simulink model "LCK"  (R2018b)
settings: Solver=FixedStepDiscrete  StartTime=0.0  StopTime=inf  FixedStep=0.01  RelTol=1e-3
PostLoadFcn:
  | if any(exist('dsrtsu_mdlpostloadfcn', 'file') ~= 0), dsrtsu_mdlpostloadfcn('Execute', bdroot); end
values from neighbouring files (symbols this model uses):
  C_DEG2RAD = 0.0175    [LCK_Macro.sldd]
  C_KPH2MPS = 0.2778    [LCK_Macro.sldd]
  C_NEARZERO = 0.0001    [LCK_Macro.sldd]
  C_ONE = 1.0    [LCK_Macro.sldd]
  C_RAD2DEG = 57.2958    [LCK_Macro.sldd]
  C_ZERO = 0.0    [LCK_Macro.sldd]
  k_accel_pedal_pos_per_speed_x : value not decoded    [LCK_LogicPara.sldd]
  k_accel_pedal_pos_per_speed_z : value not decoded    [LCK_LogicPara.sldd]
  k_brake_suprress_hold = 1000.0    [LCK_LogicPara.sldd]
  k_driver_appl_torque_filt = 50.0    [LCK_LogicPara.sldd]
  k_driver_suppression_hold_time = 3000.0    [LCK_LogicPara.sldd]
  k_hands_on_wheel_hold_msec = 500.0    [LCK_LogicPara.sldd]
  k_hands_on_wheel_torque_hi = 0.2    [LCK_LogicPara.sldd]
  k_hands_on_wheel_torque_lo = 0.15    [LCK_LogicPara.sldd]
  k_handsoff_delay_cycles = 50.0    [LCK_LogicPara.sldd]
  k_handsoff_torq_Lo_CR = 0.3    [LCK_LogicPara.sldd]
  k_handson_delay_cycles = 5.0    [LCK_LogicPara.sldd]
  k_HighAccel_suppress_hold = 3000.0    [LCK_LogicPara.sldd]
  k_HLR_suprress_hold = 3000.0    [LCK_LogicPara.sldd]
  k_hs_StrAng_CR_threshold_z : value not decoded    [LCK_LogicPara.sldd]
  k_LC_Exit_Switch = 0.0    [LCK_LogicPara.sldd]
  k_LCG_Configured = 1.0    [LCK_LogicPara.sldd]
  k_LCK_A0_Rdy2Act_UseConst = 0.0    [LCK_LogicPara.sldd]
  k_LCK_A0Fac_ActSta : value not decoded    [LCK_CtrlPara.sldd]
  k_LCK_A0Fac_DrvStm : value not decoded    [LCK_CtrlPara.sldd]
  k_LCK_A0Shift_LftCurv : value not decoded    [LCK_CtrlPara.sldd]
  k_LCK_A0Shift_RgtCurv : value not decoded    [LCK_CtrlPara.sldd]
  k_LCK_A0Shift_StraLan = 0.0    [LCK_CtrlPara.sldd]
  k_LCK_A0ShiftFac_Dy_LftCurv : value not decoded    [LCK_CtrlPara.sldd]
  k_LCK_A0ShiftFac_Dy_RgtCurv : value not decoded    [LCK_CtrlPara.sldd]
  k_LCK_A0ShiftFac_Vspd : value not decoded    [LCK_CtrlPara.sldd]
  k_LCK_accel_inhibit_thold = 35.0    [LCK_LogicPara.sldd]
  k_LCK_Active2Ready_Mask = 255.0    [LCK_LogicPara.sldd]
  k_LCK_CvatRateBks : value not decoded    [LCK_CtrlPara.sldd]
  k_LCK_CvatrBks : value not decoded    [LCK_CtrlPara.sldd]
  k_LCK_DFac_Dy : value not decoded    [LCK_CtrlPara.sldd]
  k_LCK_DFac_Dy_Curv : value not decoded    [LCK_CtrlPara.sldd]
  k_LCK_DFac_HaCurCen : value not decoded    [LCK_CtrlPara.sldd]
  k_LCK_DFac_HaCurSid : value not decoded    [LCK_CtrlPara.sldd]
  k_LCK_DFac_HadCurCen : value not decoded    [LCK_CtrlPara.sldd]
  k_LCK_DFac_HadCurSid : value not decoded    [LCK_CtrlPara.sldd]
  k_LCK_DFac_HadStrCen : value not decoded    [LCK_CtrlPara.sldd]
  k_LCK_DFac_HadStrSid : value not decoded    [LCK_CtrlPara.sldd]
  k_LCK_DFac_HaStrCen : value not decoded    [LCK_CtrlPara.sldd]
  k_LCK_DFac_HaStrSid : value not decoded    [LCK_CtrlPara.sldd]
  k_LCK_DFac_Rad : value not decoded    [LCK_CtrlPara.sldd]
  k_LCK_DFac_SA_CurCen : value not decoded    [LCK_CtrlPara.sldd]
  k_LCK_DFac_SA_CurSid : value not decoded    [LCK_CtrlPara.sldd]
  k_LCK_DFac_SA_StrCen : value not decoded    [LCK_CtrlPara.sldd]
  k_LCK_DFac_SA_StrSid : value not decoded    [LCK_CtrlPara.sldd]
  k_LCK_DFac_SS_CurCen : value not decoded    [LCK_CtrlPara.sldd]
  k_LCK_DFac_SS_CurSid : value not decoded    [LCK_CtrlPara.sldd]
  k_LCK_DFac_SS_StrCen : value not decoded    [LCK_CtrlPara.sldd]
  k_LCK_DFac_SS_StrSid : value not decoded    [LCK_CtrlPara.sldd]
  k_LCK_DFac_Vspd : value not decoded    [LCK_CtrlPara.sldd]
  k_LCK_DlyTm_DrvStim = 0.2    [LCK_CtrlPara.sldd]
  k_LCK_DTermMax = 2.0    [LCK_CtrlPara.sldd]
  k_LCK_DyBks_Curv : value not decoded    [LCK_CtrlPara.sldd]
  k_LCK_Enable_POOnly = 1.0    [LCK_LogicPara.sldd]
  k_LCK_Entry_DistBuffer = 0.1    [LCK_LogicPara.sldd]
  k_LCK_Fac_Vspd2RngThr_FalRec = 0.23    [LCK_CtrlPara.sldd]
  k_LCK_Ffw_CvatSwh = 0.0    [LCK_CtrlPara.sldd]
  k_LCK_Ffw_DyBks : value not decoded    [LCK_CtrlPara.sldd]
  k_LCK_Ffw_TimCon_CmdFlt = 0.0    [LCK_CtrlPara.sldd]
  k_LCK_FfwDeltaFac_Rad_Lft : value not decoded    [LCK_CtrlPara.sldd]
  k_LCK_FfwDeltaFac_Rad_Rgt : value not decoded    [LCK_CtrlPara.sldd]
  k_LCK_FfwDeltaFac_Vspd : value not decoded    [LCK_CtrlPara.sldd]
  k_LCK_FfwFac_CvatRate_Lft : value not decoded    [LCK_CtrlPara.sldd]
  k_LCK_FfwFac_CvatRate_Rgt : value not decoded    [LCK_CtrlPara.sldd]
  k_LCK_FfwFac_Dy : value not decoded    [LCK_CtrlPara.sldd]
  k_LCK_FfwFac_Rad_Lft : value not decoded    [LCK_CtrlPara.sldd]
  k_LCK_FfwFac_Rad_Rgt : value not decoded    [LCK_CtrlPara.sldd]
  k_LCK_FfwFac_Vspd : value not decoded    [LCK_CtrlPara.sldd]
  k_LCK_FfwTorq_Cvat : value not decoded    [LCK_CtrlPara.sldd]
  k_LCK_HAFac_ActSta : value not decoded    [LCK_CtrlPara.sldd]
  k_LCK_HAFac_DrvStm : value not decoded    [LCK_CtrlPara.sldd]
  k_LCK_HaloTime = 2000.0    [LCK_LogicPara.sldd]
  k_LCK_HaloTime_Switch = 0.0    [LCK_LogicPara.sldd]
  k_LCK_HARFac_ActSta : value not decoded    [LCK_CtrlPara.sldd]
  k_LCK_HARFac_DrvStm : value not decoded    [LCK_CtrlPara.sldd]
  k_LCK_Hed_DyBks : value not decoded    [LCK_CtrlPara.sldd]
  k_LCK_HedAngDiffX : value not decoded    [LCK_CtrlPara.sldd]
  k_LCK_HedAngRateDiffX : value not decoded    [LCK_CtrlPara.sldd]
  k_LCK_HndsOnWhel_DlyTm_Idl2Rdy = 0.0    [LCK_LogicPara.sldd]
  k_LCK_host_veh_width = 1.86    [LCK_LogicPara.sldd]
  k_LCK_Idle2Ready_Mask = 239.0    [LCK_LogicPara.sldd]
  k_LCK_Junc_SusTime = 1.0    [LCK_LogicPara.sldd]
  k_LCK_KpKdDecSlopeLmt = 10.0    [LCK_CtrlPara.sldd]
  k_LCK_KpKdIncSlopeLmt = 5.0    [LCK_CtrlPara.sldd]
  k_LCK_Lat_Ctrl_DFac_Lft = 1.0    [LCK_CtrlPara.sldd]
  k_LCK_Lat_Ctrl_DFac_Rgt = 1.05    [LCK_CtrlPara.sldd]
  k_LCK_Lat_Ctrl_Kd = 0.8    [LCK_CtrlPara.sldd]
  k_LCK_Lat_Ctrl_Ki = 0.5    [LCK_CtrlPara.sldd]
  k_LCK_Lat_Ctrl_Kp = 0.7    [LCK_CtrlPara.sldd]
  k_LCK_Lat_Ctrl_Kp_NearGain = 0.7    [LCK_CtrlPara.sldd]
  k_LCK_Lat_Ctrl_PFac_Lft = 1.0    [LCK_CtrlPara.sldd]
  k_LCK_Lat_Ctrl_PFac_Rgt = 1.05    [LCK_CtrlPara.sldd]
  k_LCK_Lat_Ctrl_TimCon_CmdFlt = 5.0    [LCK_CtrlPara.sldd]
  k_LCK_Lat_DFac_Rad : value not decoded    [LCK_CtrlPara.sldd]
  k_LCK_Lat_DFac_SS_Cur : value not decoded    [LCK_CtrlPara.sldd]
  k_LCK_Lat_DFac_SS_Str : value not decoded    [LCK_CtrlPara.sldd]
  k_LCK_Lat_DFac_Vspd : value not decoded    [LCK_CtrlPara.sldd]
  k_LCK_Lat_DyBks : value not decoded    [LCK_CtrlPara.sldd]
  k_LCK_Lat_IFac_Rad : value not decoded    [LCK_CtrlPara.sldd]
  k_LCK_Lat_IFac_Vspd : value not decoded    [LCK_CtrlPara.sldd]
  k_LCK_Lat_ILmtFac_Dy_CurvLan : value not decoded    [LCK_CtrlPara.sldd]
  k_LCK_Lat_ILmtFac_Dy_StraLan : value not decoded    [LCK_CtrlPara.sldd]
  k_LCK_Lat_ILmtFac_Rad : value not decoded    [LCK_CtrlPara.sldd]
  k_LCK_Lat_ILmtFac_Rad_NearGain = 1.0    [LCK_CtrlPara.sldd]
  k_LCK_Lat_ILmtFac_Vspd_CurvLan : value not decoded    [LCK_CtrlPara.sldd]
  k_LCK_Lat_ILmtFac_Vspd_StraLan : value not decoded    [LCK_CtrlPara.sldd]
  k_LCK_Lat_ITermLmt_Dy = 1.0    [LCK_CtrlPara.sldd]
  k_LCK_Lat_KpKdDecSlopeLmt = 10.0    [LCK_CtrlPara.sldd]
  k_LCK_Lat_KpKdIncSlopeLmt = 10.0    [LCK_CtrlPara.sldd]
  k_LCK_Lat_PFac_Dy_InnLftCur : value not decoded    [LCK_CtrlPara.sldd]
  k_LCK_Lat_PFac_Dy_InnRgtCur : value not decoded    [LCK_CtrlPara.sldd]
  k_LCK_Lat_PFac_Dy_OutLftCur : value not decoded    [LCK_CtrlPara.sldd]
  k_LCK_Lat_PFac_Dy_OutRgtCur : value not decoded    [LCK_CtrlPara.sldd]
  k_LCK_Lat_PFac_Dy_Str : value not decoded    [LCK_CtrlPara.sldd]
  k_LCK_Lat_PFac_Rad : value not decoded    [LCK_CtrlPara.sldd]
  ... (+153 more)
undefined symbols (not defined in the file or in its folder): k_LCK_CurvBks, K_LCK_SPA0A1A2_LMRngCmp_y
libraries: LateralControl_fcns_lib x59, simulink x24
(part 42 of 47)

== system LCK/Lateral_Control_Module/Adas_Lateral_Control_LCK_Core/Module 9/Module 0/Definition Fac 4 ==
  Steer_Ang : Inport
  Cen_Flag : Inport  Port=2
  Str_Flag : Inport  Port=3
  Abs1 : Abs
  Switch{19..24} (6 alike) : Switch  Criteria=u2 > Threshold
  k_LCK_DFac_SA_CurCen : Lookup_n-D  NumberOfTableDimensions=1  BreakpointsForDimension1=k_LCK_StrAngBks  IndexSearchMethod=Linear search  Table=k_LCK_DFac_SA_CurCen  ExtrapMethod=Clip  InternalRulePriority=Speed  RndMeth=Simplest  InputSameDT=on
  k_LCK_DFac_SA_CurSid : Lookup_n-D  NumberOfTableDimensions=1  BreakpointsForDimension1=k_LCK_StrAngBks  IndexSearchMethod=Linear search  Table=k_LCK_DFac_SA_CurSid  ExtrapMethod=Clip  InternalRulePriority=Speed  RndMeth=Simplest  InputSameDT=on
  k_LCK_DFac_SA_StrCen : Lookup_n-D  NumberOfTableDimensions=1  BreakpointsForDimension1=k_LCK_StrAngBks  IndexSearchMethod=Linear search  Table=k_LCK_DFac_SA_StrCen  ExtrapMethod=Clip  InternalRulePriority=Speed  RndMeth=Simplest  InputSameDT=on
  k_LCK_DFac_SA_StrSid : Lookup_n-D  NumberOfTableDimensions=1  BreakpointsForDimension1=k_LCK_StrAngBks  IndexSearchMethod=Linear search  Table=k_LCK_DFac_SA_StrSid  ExtrapMethod=Clip  InternalRulePriority=Speed  RndMeth=Simplest  InputSameDT=on
  k_LCK_PFac_SA_CurCen : Lookup_n-D  NumberOfTableDimensions=1  BreakpointsForDimension1=k_LCK_StrAngBks  IndexSearchMethod=Linear search  Table=k_LCK_PFac_SA_CurCen  ExtrapMethod=Clip  InternalRulePriority=Speed  RndMeth=Simplest  InputSameDT=on
  k_LCK_PFac_SA_CurSid : Lookup_n-D  NumberOfTableDimensions=1  BreakpointsForDimension1=k_LCK_StrAngBks  IndexSearchMethod=Linear search  Table=k_LCK_PFac_SA_CurSid  ExtrapMethod=Clip  InternalRulePriority=Speed  RndMeth=Simplest  InputSameDT=on
  k_LCK_PFac_SA_StrCen : Lookup_n-D  NumberOfTableDimensions=1  BreakpointsForDimension1=k_LCK_StrAngBks  IndexSearchMethod=Linear search  Table=k_LCK_PFac_SA_StrCen  ExtrapMethod=Clip  InternalRulePriority=Speed  RndMeth=Simplest  InputSameDT=on
  k_LCK_PFac_SA_StrSid : Lookup_n-D  NumberOfTableDimensions=1  BreakpointsForDimension1=k_LCK_StrAngBks  IndexSearchMethod=Linear search  Table=k_LCK_PFac_SA_StrSid  ExtrapMethod=Clip  InternalRulePriority=Speed  RndMeth=Simplest  InputSameDT=on
  LatCtrl_PFac_StrAng : Outport
  LatCtrl_DFac_StrAng : Outport  Port=2
  wires:
  Switch19/1 -> Switch24/1
  Switch22/1 -> Switch24/3
  Steer_Ang/1 -> Abs1/1
  k_LCK_DFac_SA_StrCen/1 -> Switch21/1
  k_LCK_DFac_SA_CurSid/1 -> Switch23/3
  k_LCK_PFac_SA_StrSid/1 -> Switch19/3
  k_LCK_DFac_SA_CurCen/1 -> Switch23/1
  k_LCK_PFac_SA_StrCen/1 -> Switch19/1
  k_LCK_DFac_SA_StrSid/1 -> Switch21/3
  k_LCK_PFac_SA_CurCen/1 -> Switch22/1
  k_LCK_PFac_SA_CurSid/1 -> Switch22/3
  Cen_Flag/1 -> Switch21/2, Switch23/2, Switch22/2, Switch19/2
  Switch21/1 -> Switch20/1
  Switch23/1 -> Switch20/3
  Switch20/1 -> LatCtrl_DFac_StrAng/1
  Abs1/1 -> k_LCK_PFac_SA_CurSid/1, k_LCK_DFac_SA_StrCen/1, k_LCK_DFac_SA_StrSid/1, k_LCK_DFac_SA_CurCen/1, k_LCK_DFac_SA_CurSid/1, k_LCK_PFac_SA_CurCen/1, k_LCK_PFac_SA_StrSid/1, k_LCK_PFac_SA_StrCen/1
  Str_Flag/1 -> Switch20/2, Switch24/2
  Switch24/1 -> LatCtrl_PFac_StrAng/1

== system LCK/Lateral_Control_Module/Adas_Lateral_Control_LCK_Core/Module 9/Module 0/Definition Fac 5 ==
  Steer_Spd : Inport
  Cen_Flag : Inport  Port=2
  Str_Flag : Inport  Port=3
  Abs4 : Abs
  Switch{13..18} (6 alike) : Switch  Criteria=u2 > Threshold
  k_LCK_DFac_SS_CurCen : Lookup_n-D  NumberOfTableDimensions=1  BreakpointsForDimension1=k_LCK_StrSpdBks  IndexSearchMethod=Linear search  Table=k_LCK_DFac_SS_CurCen  ExtrapMethod=Clip  InternalRulePriority=Speed  RndMeth=Simplest  InputSameDT=on
  k_LCK_DFac_SS_CurSid : Lookup_n-D  NumberOfTableDimensions=1  BreakpointsForDimension1=k_LCK_StrSpdBks  IndexSearchMethod=Linear search  Table=k_LCK_DFac_SS_CurSid  ExtrapMethod=Clip  InternalRulePriority=Speed  RndMeth=Simplest  InputSameDT=on
  k_LCK_DFac_SS_StrCen : Lookup_n-D  NumberOfTableDimensions=1  BreakpointsForDimension1=k_LCK_StrSpdBks  IndexSearchMethod=Linear search  Table=k_LCK_DFac_SS_StrCen  ExtrapMethod=Clip  InternalRulePriority=Speed  RndMeth=Simplest  InputSameDT=on
  k_LCK_DFac_SS_StrSid : Lookup_n-D  NumberOfTableDimensions=1  BreakpointsForDimension1=k_LCK_StrSpdBks  IndexSearchMethod=Linear search  Table=k_LCK_DFac_SS_StrSid  ExtrapMethod=Clip  InternalRulePriority=Speed  RndMeth=Simplest  InputSameDT=on
  k_LCK_PFac_SS_CurCen : Lookup_n-D  NumberOfTableDimensions=1  BreakpointsForDimension1=k_LCK_StrSpdBks  IndexSearchMethod=Linear search  Table=k_LCK_PFac_SS_CurCen  ExtrapMethod=Clip  InternalRulePriority=Speed  RndMeth=Simplest  InputSameDT=on
  k_LCK_PFac_SS_CurSid : Lookup_n-D  NumberOfTableDimensions=1  BreakpointsForDimension1=k_LCK_StrSpdBks  IndexSearchMethod=Linear search  Table=k_LCK_PFac_SS_CurSid  ExtrapMethod=Clip  InternalRulePriority=Speed  RndMeth=Simplest  InputSameDT=on
  k_LCK_PFac_SS_StrCen : Lookup_n-D  NumberOfTableDimensions=1  BreakpointsForDimension1=k_LCK_StrSpdBks  IndexSearchMethod=Linear search  Table=k_LCK_PFac_SS_StrCen  ExtrapMethod=Clip  InternalRulePriority=Speed  RndMeth=Simplest  InputSameDT=on
  k_LCK_PFac_SS_StrSid : Lookup_n-D  NumberOfTableDimensions=1  BreakpointsForDimension1=k_LCK_StrSpdBks  IndexSearchMethod=Linear search  Table=k_LCK_PFac_SS_StrSid  ExtrapMethod=Clip  InternalRulePriority=Speed  RndMeth=Simplest  InputSameDT=on
  LatCtrl_PFac_StrSpd : Outport
  LatCtrl_DFac_StrSpd : Outport  Port=2
  wires:
  Abs4/1 -> k_LCK_PFac_SS_StrCen/1, k_LCK_PFac_SS_CurCen/1, k_LCK_PFac_SS_CurSid/1, k_LCK_DFac_SS_StrCen/1, k_LCK_DFac_SS_StrSid/1, k_LCK_DFac_SS_CurSid/1, k_LCK_DFac_SS_CurCen/1, k_LCK_PFac_SS_StrSid/1
  Str_Flag/1 -> Switch14/2, Switch18/2
  Switch18/1 -> LatCtrl_PFac_StrSpd/1
  Steer_Spd/1 -> Abs4/1
  k_LCK_PFac_SS_StrCen/1 -> Switch13/1
  k_LCK_DFac_SS_CurCen/1 -> Switch17/1
  Switch15/1 -> Switch14/1
  Switch17/1 -> Switch14/3
  Switch14/1 -> LatCtrl_DFac_StrSpd/1
  k_LCK_PFac_SS_CurSid/1 -> Switch16/3
  k_LCK_PFac_SS_StrSid/1 -> Switch13/3
  k_LCK_PFac_SS_CurCen/1 -> Switch16/1
  Cen_Flag/1 -> Switch16/2, Switch17/2, Switch15/2, Switch13/2
  k_LCK_DFac_SS_CurSid/1 -> Switch17/3
  k_LCK_DFac_SS_StrCen/1 -> Switch15/1
  Switch13/1 -> Switch18/1
  k_LCK_DFac_SS_StrSid/1 -> Switch15/3
  Switch16/1 -> Switch18/3

== system LCK/Lateral_Control_Module/Adas_Lateral_Control_LCK_Core/Module 9/Module 0/Definition Fac 6 ==
  Str_Flag : Inport
  Dy_0 : Inport  Port=2
  Abs : Abs
  Switch27 : Switch  Criteria=u2 > Threshold
  Switch28 : Switch  Criteria=u2 > Threshold
  k_LCK_DFac_Dy : Lookup_n-D  NumberOfTableDimensions=1  BreakpointsForDimension1=k_LCK_Hed_DyBks  IndexSearchMethod=Linear search  Table=k_LCK_DFac_Dy  ExtrapMethod=Clip  InternalRulePriority=Speed  RndMeth=Simplest  InputSameDT=on
  k_LCK_DFac_Dy_Curv : Lookup_n-D  NumberOfTableDimensions=1  BreakpointsForDimension1=k_LCK_Hed_DyBks  IndexSearchMethod=Linear search  Table=k_LCK_DFac_Dy_Curv  ExtrapMethod=Clip  InternalRulePriority=Speed  RndMeth=Simplest  InputSameDT=on
  k_LCK_PFac_Dy : Lookup_n-D  NumberOfTableDimensions=1  BreakpointsForDimension1=k_LCK_Hed_DyBks  IndexSearchMethod=Linear search  Table=k_LCK_PFac_Dy  ExtrapMethod=Clip  InternalRulePriority=Speed  RndMeth=Simplest  InputSameDT=on
  k_LCK_PFac_Dy_Curv : Lookup_n-D  NumberOfTableDimensions=1  BreakpointsForDimension1=k_LCK_Hed_DyBks  IndexSearchMethod=Linear search  Table=k_LCK_PFac_Dy_Curv  ExtrapMethod=Clip  InternalRulePriority=Speed  RndMeth=Simplest  InputSameDT=on
  LatCtrl_PFac_Dy : Outport
  LatCtrl_DFac_Dy : Outport  Port=2
  wires:
  k_LCK_PFac_Dy_Curv/1 -> Switch27/3
  Switch27/1 -> LatCtrl_PFac_Dy/1
  k_LCK_PFac_Dy/1 -> Switch27/1
  Str_Flag/1 -> Switch28/2, Switch27/2
  k_LCK_DFac_Dy_Curv/1 -> Switch28/3
  k_LCK_DFac_Dy/1 -> Switch28/1
  Switch28/1 -> LatCtrl_DFac_Dy/1
  Dy_0/1 -> Abs/1
  Abs/1 -> k_LCK_PFac_Dy_Curv/1, k_LCK_DFac_Dy_Curv/1, k_LCK_DFac_Dy/1, k_LCK_PFac_Dy/1

== system LCK/Lateral_Control_Module/Adas_Lateral_Control_LCK_Core/Module 9/Module 0/Definition Fac 7 ==
  Vspd : Inport
  k_LCK_DFac_Vspd : Lookup_n-D  NumberOfTableDimensions=1  BreakpointsForDimension1=k_LCK_VspdBks  IndexSearchMethod=Linear search  Table=k_LCK_DFac_Vspd  ExtrapMethod=Clip  InternalRulePriority=Speed  RndMeth=Simplest  InputSameDT=on
  k_LCK_PFac_Vspd : Lookup_n-D  NumberOfTableDimensions=1  BreakpointsForDimension1=k_LCK_VspdBks  IndexSearchMethod=Linear search  Table=k_LCK_PFac_Vspd  ExtrapMethod=Clip  InternalRulePriority=Speed  RndMeth=Simplest  InputSameDT=on
  LatCtrl_PFac_Vspd : Outport
  LatCtrl_DFac_Vspd : Outport  Port=2
  wires:
  k_LCK_PFac_Vspd/1 -> LatCtrl_PFac_Vspd/1
  Vspd/1 -> k_LCK_DFac_Vspd/1, k_LCK_PFac_Vspd/1
  k_LCK_DFac_Vspd/1 -> LatCtrl_DFac_Vspd/1
